simulink model "TDPC_energydomain"  (R2019b)
settings: Solver=ode4  StartTime=0.0  StopTime=20  FixedStep=0.0001  MaxStep=0.1  MinStep=0.001  RelTol=1e-6  AbsTol=1e-6
libraries: simulink x2
settings Model: Creator=meetn  LastModifiedBy=manth
settings SolverCC: ZeroCrossAlgorithm=Adaptive  AlgebraicLoopSolver=LineSearch
settings DebuggingCC: UnderSpecifiedDimensionMsg=warning

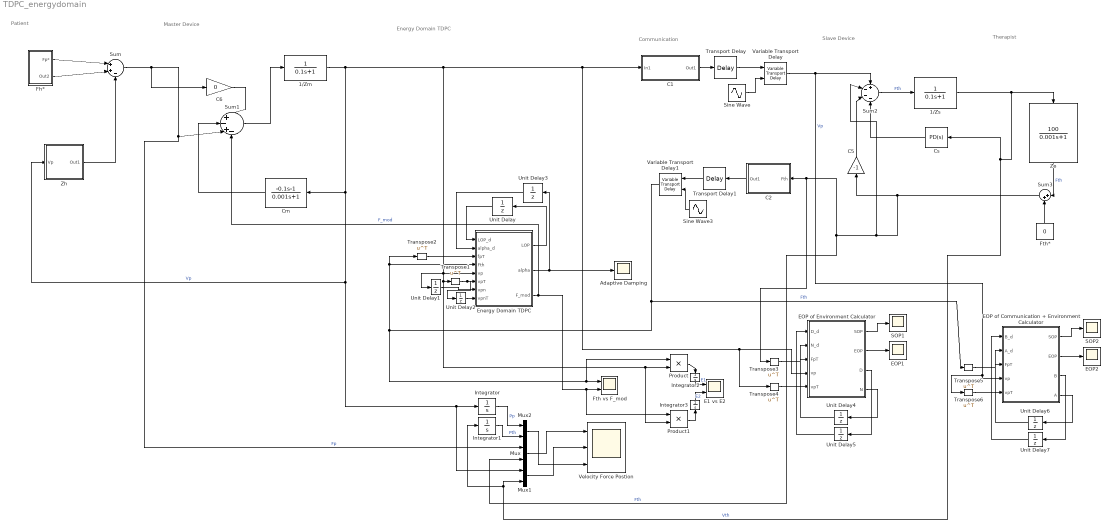
== system TDPC_energydomain ==
  note: Energy Domain TDPC
  note: Communication
  note: Slave Device
  note: Therapist
  note: Master Device
  note: Patient
  1/Zm : TransferFcn  Denominator=[0.1 1]
  1/Zs : TransferFcn  Denominator=[0.1 1]
  Adaptive Damping : Scope
  C1 : Subsystem
  C2 : Subsystem
  "C5 " : Gain  Gain=-1
  "C6 " : Gain  Gain=0
  Cm : TransferFcn  Numerator=[-0.1 -1]  Denominator=[0.001 1]
  Cs : simulink/Continuous/PID Controller  Controller=PD  Form=Parallel  TimeDomain=Continuous-time  SampleTime=-1  IntegratorMethod=Forward Euler  FilterMethod=Forward Euler  ControllerParametersSource=internal  P=1000  I=1  D=1  UseFilter=on  N=1000  TunerSelectOption=Transfer Function Based (PID Tuner App)  InitialConditionSource=internal  InitialConditionForIntegrator=0  InitialConditionForFilter=0  DifferentiatorICPrevScaledInput=0  ExternalReset=none  TrackingMode=off  Kt=1  LimitOutput=off  UpperSaturationLimit=inf  LowerSaturationLimit=-inf  LinearizeAsGain=on  AntiWindupMode=none  Kb=1  POutMin=[]  POutMax=[]  IOutMin=[]  IOutMax=[]  DOutMin=[]  DOutMax=[]  NOutMin=[]  NOutMax=[]  SumOutMin=[]  SumOutMax=[]  SaturationOutMin=[]  SaturationOutMax=[]  PParamMin=[]  PParamMax=[]  IParamMin=[]  IParamMax=[]  DParamMin=[]  DParamMax=[]  NParamMin=[]  NParamMax=[]  KbParamMin=[]  KbParamMax=[]  KtParamMin=[]  KtParamMax=[]  KbOutMin=[]  KbOutMax=[]  KtOutMin=[]  KtOutMax=[]  IntegratorOutMin=[]  IntegratorOutMax=[]  FilterOutMin=[]  FilterOutMax=[]  SumI1OutMin=[]  SumI1OutMax=[]  SumI2OutMin=[]  SumI2OutMax=[]  SumI3OutMin=[]  SumI3OutMax=[]  SumI4OutMin=[]  SumI4OutMax=[]  SumDOutMin=[]  SumDOutMax=[]  DifferentiatorOutMin=[]  DifferentiatorOutMax=[]  FilterDiffOutCoefMin=[]  FilterDiffOutCoefMax=[]  ReciprocalOutMin=[]  ReciprocalOutMax=[]  SumDenOutMin=[]  SumDenOutMax=[]  SumNumOutMin=[]  SumNumOutMax=[]  DivideOutMin=[]  DivideOutMax=[]  IntegratorContinuousStateAttributes=''  IntegratorStateMustResolveToSignalObject=off  IntegratorRTWStateStorageClass=Auto  FilterContinuousStateAttributes=''  FilterStateMustResolveToSignalObject=off  FilterRTWStateStorageClass=Auto  ParallelPVariant=InternalParameters  IdealPVariant=Disabled  IVariant=Disabled  DVariant=InternalParameters  IntegratorVariant=Disabled  SatVariant=Disabled  AWVariant=Disabled  PCopyVariant=Disabled  TRVariant=Disabled  FdbkBlocksVariant=Forward  IdealPFdbkVariant=Disabled  SatFdbkVariant=Disabled  DerivativeFilterVariant=ContFilter  NVariant=InternalParameters  NCopyVariant=Disabled  FilterICVariant=InternalICsFilter  IntegratorICVariant=Disabled  ExternalResetVariant=Disabled  TRSumVariant=Passthrough  SumFdbkVariant=Disabled  SumVariant=Sum_PD
  E1 vs E2 : Scope  NumInputPorts=2
  EOP of Communication + Environment Calculator : MATLAB Function  TreatAsAtomicUnit=on
  EOP of Environment Calculator : MATLAB Function  TreatAsAtomicUnit=on
  EOP1 : Scope
  EOP2 : Scope
  Energy Domain TDPC : MATLAB Function  TreatAsAtomicUnit=on
  Fh* : Subsystem
  Fth vs F_mod : Scope  NumInputPorts=2
  Fth* : Constant  Value=0  OutDataTypeStr=Inherit: Inherit via back propagation
  Integrator{,1..3} (4 alike) : Integrator
  Mux : Mux  Inputs=2
  Mux1 : Mux  Inputs=2
  Mux2 : Mux  Inputs=2
  Product : Product
  Product1 : Product
  SOP1 : Scope
  SOP2 : Scope
  Sine Wave : Sin  Amplitude=0.02  Frequency=12  SampleTime=0
  Sine Wave3 : Sin  Amplitude=0.02  Frequency=12  SampleTime=0
  Sum : Sum  Inputs=|++-
  Sum1 : Sum  Inputs=|+-+-
  Sum2 : Sum  Inputs=+---
  Sum3 : Sum  Inputs=|++
  Transport Delay : TransportDelay  DelayTime=0.1  PadeOrder=3
  Transport Delay1 : TransportDelay  DelayTime=0.1  PadeOrder=3
  Transpose{1..6} (6 alike) : Math  Operator=transpose  SignedPower=off  SaturateOnIntegerOverflow=on
  Unit Delay{,1..7} (8 alike) : UnitDelay  SampleTime=-1  HasFrameUpgradeWarning=on
  Variable Transport Delay : VariableTransportDelay  PadeOrder=3
  Variable Transport Delay1 : VariableTransportDelay  PadeOrder=3
  Velocity Force Postion : Scope  NumInputPorts=3
  Ze : TransferFcn  Numerator=[100]  Denominator=[0.001 1]
  Zh : Subsystem
  wires:
  "C6 "/1 -> Sum1/1
  Cs/1 -> Sum2/4
  Ze/1 -> Sum3/1  "Fth"
  Sum1/1 -> 1/Zm/1
  Fth*/1 -> Sum3/2
  1/Zs/1 -> Ze/1, Cs/1, Integrator1/1, Mux1/2  "Vth"
  Sum2/1 -> 1/Zs/1  "Fth"
  Sum/1 -> "C6 "/1, Mux/1, Sum1/3  "Fp"
  "C5 "/1 -> Sum2/3
  Cm/1 -> Sum1/2
  Sum3/1 -> Sum2/2, Transpose3/1, C2/1(Fth), Mux/2, "C5 "/1  "Fth"
  1/Zm/1 -> Mux1/1, Integrator/1, Zh/1(Vp), Cm/1, Transpose1/1, Product1/2, Product/2, Unit Delay1/1, Energy Domain TDPC/5(vp), Transpose4/1, EOP of Environment Calculator/4(vp), C1/1(In1)  "Vp"
  Mux/1 -> Velocity Force Postion/1
  Mux1/1 -> Velocity Force Postion/2
  Unit Delay/1 -> Energy Domain TDPC/1(LOP_d)
  Energy Domain TDPC/1(LOP) -> Unit Delay/1
  Unit Delay2/1 -> Energy Domain TDPC/8(vpnT)
  Energy Domain TDPC/2(alpha) -> Unit Delay3/1, Adaptive Damping/1
  Unit Delay3/1 -> Energy Domain TDPC/2(alpha_d)
  Energy Domain TDPC/3(F_mod) -> Sum1/4, Product1/1, Fth vs F_mod/2  "F_mod"
  Variable Transport Delay1/1 -> Transpose2/1, Energy Domain TDPC/4(Fth), Product/1, Fth vs F_mod/1, Transpose5/1  "Fth"
  Mux2/1 -> Velocity Force Postion/3
  Integrator/1 -> Mux2/1  "Pp"
  Integrator1/1 -> Mux2/2  "Pth"
  Sine Wave/1 -> Variable Transport Delay/2
  Transport Delay/1 -> Variable Transport Delay/1
  C1/1(Out1) -> Transport Delay/1
  Sine Wave3/1 -> Variable Transport Delay1/2
  Transport Delay1/1 -> Variable Transport Delay1/1
  C2/1(Out1) -> Transport Delay1/1
  Fh*/1(Fp*) -> Sum/1
  Fh*/2(Out2) -> Sum/2
  Zh/1(Out1) -> Sum/3
  Transpose1/1 -> Unit Delay2/1, Energy Domain TDPC/6(vpT)
  Unit Delay1/1 -> Energy Domain TDPC/7(vpn)
  Transpose2/1 -> Energy Domain TDPC/3(fpT)
  Product1/1 -> Integrator3/1
  Integrator3/1 -> E1 vs E2/2  "E2"
  Integrator2/1 -> E1 vs E2/1  "E1"
  Product/1 -> Integrator2/1
  EOP of Environment Calculator/4(N) -> Unit Delay4/1
  Unit Delay4/1 -> EOP of Environment Calculator/2(N_d)
  EOP of Environment Calculator/3(D) -> Unit Delay5/1
  Unit Delay5/1 -> EOP of Environment Calculator/1(D_d)
  Transpose3/1 -> EOP of Environment Calculator/3(FpT)
  Transpose4/1 -> EOP of Environment Calculator/5(vpT)
  EOP of Environment Calculator/1(SOP) -> SOP1/1
  EOP of Environment Calculator/2(EOP) -> EOP1/1
  EOP of Communication + Environment Calculator/4(A) -> Unit Delay6/1
  Unit Delay7/1 -> EOP of Communication + Environment Calculator/1(B_d)
  Transpose6/1 -> EOP of Communication + Environment Calculator/5(vpT)
  EOP of Communication + Environment Calculator/2(EOP) -> EOP2/1
  Transpose5/1 -> EOP of Communication + Environment Calculator/3(FpT)
  Variable Transport Delay/1 -> Transpose6/1, EOP of Communication + Environment Calculator/4(vp), Sum2/1  "Vp"
  EOP of Communication + Environment Calculator/1(SOP) -> SOP2/1
  EOP of Communication + Environment Calculator/3(B) -> Unit Delay7/1
  Unit Delay6/1 -> EOP of Communication + Environment Calculator/2(A_d)

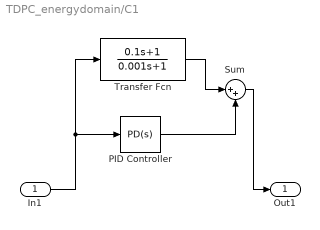
== system TDPC_energydomain/C1 ==
  In1 : Inport
  PID Controller : simulink/Continuous/PID Controller  Controller=PD  Form=Parallel  TimeDomain=Continuous-time  SampleTime=-1  IntegratorMethod=Forward Euler  FilterMethod=Forward Euler  ControllerParametersSource=internal  P=1000  I=1  D=1  UseFilter=on  N=1000  TunerSelectOption=Transfer Function Based (PID Tuner App)  InitialConditionSource=internal  InitialConditionForIntegrator=0  InitialConditionForFilter=0  DifferentiatorICPrevScaledInput=0  ExternalReset=none  TrackingMode=off  Kt=1  LimitOutput=off  UpperSaturationLimit=inf  LowerSaturationLimit=-inf  LinearizeAsGain=on  AntiWindupMode=none  Kb=1  POutMin=[]  POutMax=[]  IOutMin=[]  IOutMax=[]  DOutMin=[]  DOutMax=[]  NOutMin=[]  NOutMax=[]  SumOutMin=[]  SumOutMax=[]  SaturationOutMin=[]  SaturationOutMax=[]  PParamMin=[]  PParamMax=[]  IParamMin=[]  IParamMax=[]  DParamMin=[]  DParamMax=[]  NParamMin=[]  NParamMax=[]  KbParamMin=[]  KbParamMax=[]  KtParamMin=[]  KtParamMax=[]  KbOutMin=[]  KbOutMax=[]  KtOutMin=[]  KtOutMax=[]  IntegratorOutMin=[]  IntegratorOutMax=[]  FilterOutMin=[]  FilterOutMax=[]  SumI1OutMin=[]  SumI1OutMax=[]  SumI2OutMin=[]  SumI2OutMax=[]  SumI3OutMin=[]  SumI3OutMax=[]  SumI4OutMin=[]  SumI4OutMax=[]  SumDOutMin=[]  SumDOutMax=[]  DifferentiatorOutMin=[]  DifferentiatorOutMax=[]  FilterDiffOutCoefMin=[]  FilterDiffOutCoefMax=[]  ReciprocalOutMin=[]  ReciprocalOutMax=[]  SumDenOutMin=[]  SumDenOutMax=[]  SumNumOutMin=[]  SumNumOutMax=[]  DivideOutMin=[]  DivideOutMax=[]  IntegratorContinuousStateAttributes=''  IntegratorStateMustResolveToSignalObject=off  IntegratorRTWStateStorageClass=Auto  FilterContinuousStateAttributes=''  FilterStateMustResolveToSignalObject=off  FilterRTWStateStorageClass=Auto  ParallelPVariant=InternalParameters  IdealPVariant=Disabled  IVariant=Disabled  DVariant=InternalParameters  IntegratorVariant=Disabled  SatVariant=Disabled  AWVariant=Disabled  PCopyVariant=Disabled  TRVariant=Disabled  FdbkBlocksVariant=Forward  IdealPFdbkVariant=Disabled  SatFdbkVariant=Disabled  DerivativeFilterVariant=ContFilter  NVariant=InternalParameters  NCopyVariant=Disabled  FilterICVariant=InternalICsFilter  IntegratorICVariant=Disabled  ExternalResetVariant=Disabled  TRSumVariant=Passthrough  SumFdbkVariant=Disabled  SumVariant=Sum_PD
  Sum : Sum  Inputs=|++
  Transfer Fcn : TransferFcn  Numerator=[0.1 1]  Denominator=[0.001 1]
  Out1 : Outport
  wires:
  In1/1 -> PID Controller/1, Transfer Fcn/1
  Transfer Fcn/1 -> Sum/1
  PID Controller/1 -> Sum/2
  Sum/1 -> Out1/1

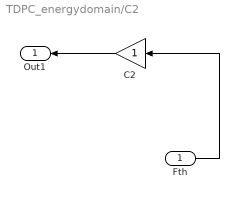
== system TDPC_energydomain/C2 ==
  Fth : Inport
  C2 : Gain
  Out1 : Outport
  wires:
  Fth/1 -> C2/1
  C2/1 -> Out1/1

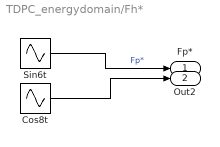
== system TDPC_energydomain/Fh* ==
  Cos8t : Sin  Frequency=8  Phase=pi/2  SampleTime=0
  Sin6t : Sin  Frequency=6  SampleTime=0
  Fp* : Outport
  Out2 : Outport  Port=2
  wires:
  Sin6t/1 -> Fp*/1  "Fp*"
  Cos8t/1 -> Out2/1

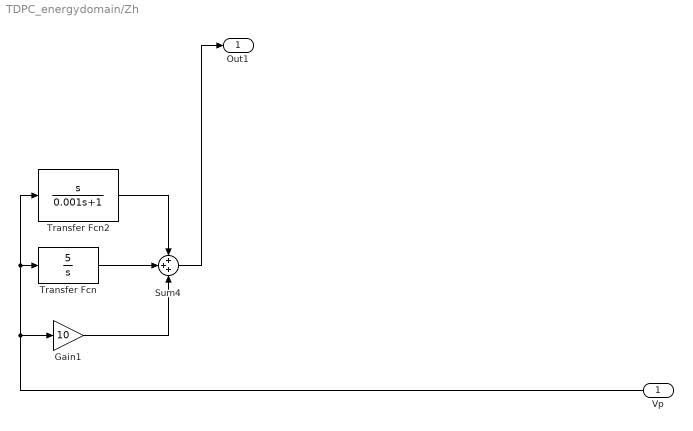
== system TDPC_energydomain/Zh ==
  Vp : Inport
  Gain1 : Gain  Gain=10
  Sum4 : Sum  Inputs=3
  Transfer Fcn : TransferFcn  Numerator=[5]  Denominator=[1 0]
  Transfer Fcn2 : TransferFcn  Numerator=[1 0]  Denominator=[0.001 1]
  Out1 : Outport
  wires:
  Vp/1 -> Gain1/1, Transfer Fcn/1, Transfer Fcn2/1
  Sum4/1 -> Out1/1
  Transfer Fcn/1 -> Sum4/2
  Transfer Fcn2/1 -> Sum4/1
  Gain1/1 -> Sum4/3

== matlab function TDPC_energydomain/EOP of Environment Calculator ==
  data: D_d input; N_d input; SOP output; EOP output; FpT input; vp input; vpT input; D output; N output
function [SOP,EOP,D,N] = EOP_Calculator(D_d,N_d,FpT,vp,vpT)

N=N_d+0.001*(FpT*vp);
D=D_d+0.001*(vpT*vp);
 
SOP=N/D;
 
EOP=-SOP;

== matlab function TDPC_energydomain/Energy Domain TDPC ==
  data: LOP_d input; alpha_d input; LOP output; alpha output; fpT input; Fth input; F_mod output; vp input; vpT input; vpn input; vpnT input
function [LOP,alpha, F_mod] = Stabilizer(LOP_d,alpha_d,fpT,Fth,vp,vpT,vpn,vpnT)

PL = (fpT*vp);
in2 = (alpha_d*vpnT*vpn);
LOP = LOP_d+(0.001*(PL+in2));

if LOP>=0
    alpha = 0;
else 
    alpha=(-LOP)/(0.001*vpT*vp)+0.00001;
end

F_mod= Fth+(alpha*vp)+0.00001;

== matlab function TDPC_energydomain/EOP of Communication + Environment Calculator ==
  data: B_d input; A_d input; SOP output; EOP output; FpT input; vp input; vpT input; B output; A output
function [SOP,EOP,B,A] = EOP_Calculator(B_d,A_d,FpT,vp,vpT)

A=A_d+0.001*(FpT*vp);
B=B_d+0.001*(vpT*vp);
 
SOP=A/B;
 
EOP=-SOP;
